simulink model "mpu6050"  (R2023b)
settings: Solver=FixedStepAuto  StartTime=0.0  StopTime=100.0  RelTol=1e-3
undefined symbols (not defined in the file): f
libraries: svdutilitieslib x1, instrumentlib x1, vrlib x1
settings Model: ExtModeTrigDuration=2  Creator=VASU  LastModifiedBy=VASU
settings OptimizationCC: EnhancedBackFolding=on  PassReuseOutputArgsAs=Individual arguments  ZeroExternalMemoryAtStartup=off  ZeroInternalMemoryAtStartup=off  MaxStackSize=64  OptimizeBlockOrder=speed  DifferentSizesBufferReuse=on  OptimizationCustomize=off  EfficientTunableParamExpr=on
settings DebuggingCC: ParameterPrecisionLossMsg=none  ParameterTunabilityLossMsg=error
settings HardwareCC: ProdBitPerPointer=32  ProdBitPerSizeT=32  ProdBitPerPtrDiffT=32  ProdLargestAtomicInteger=Long  ProdLargestAtomicFloat=Double  ProdWordSize=32  ProdHWDeviceType=ARM Compatible->ARM Cortex  UseEmbeddedCoderFeatures=off  UseSimulinkCoderFeatures=off
settings SFSimCC: MATLABDynamicMemAlloc=off
settings RTWCC: Description=Embedded Coder  SystemTargetFile=ert.tlc  HardwareBoard=ESP32-WROOM(Arduino Compatible)  TLCOptions="-aInlineSetEventsForThisBaseRateFcn=TLC_FALSE -aSuppressMultiTaskScheduler=TLC_FALSE  -aRateBasedStepFcn=0"  TemplateMakefile=ert_default_tmf  Toolchain=ESP32
settings CodeAppCC: ForceParamTrailComments=on  IgnoreCustomStorageClasses=off  OperatorAnnotations=on  SimulinkDataObjDesc=on  SFDataObjDesc=on  InsertBlockDesc=on
settings ERTTargetCC: SupportContinuousTime=on  SupportNonInlinedSFcns=on  SupportVariableSizeSignals=on  ExtModeTransport=3  ExtModeStaticAlloc=on  ExtModeAutomaticAllocSize=off  ExtModeStaticAllocSize=65536  ExtModeMexFile=ext_xcp  ExtModeIntrfLevel=Level2 - Open

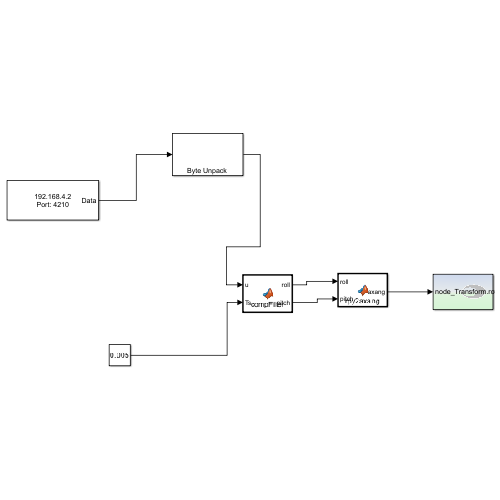
[thumbnail: Simulink's stored preview of the top-level diagram]
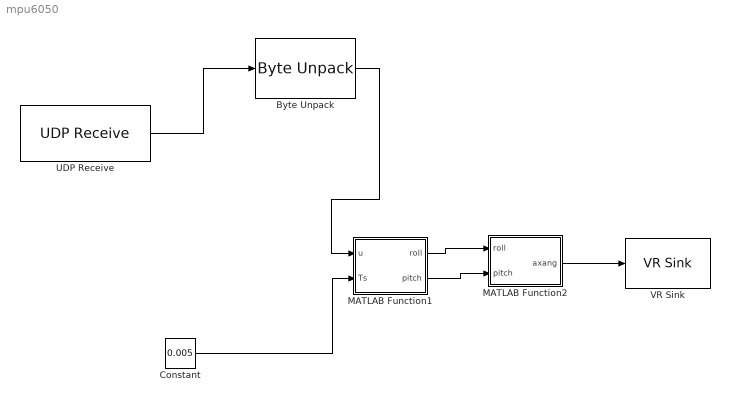
== system mpu6050 ==
  Byte Unpack : svdutilitieslib/Byte Unpack  dimensions={[6,1]}  datatypes={'single'}  byteAlign=4  blockPlatform=arduinoert
  Constant : Constant  Value=0.005  OutDataTypeStr=single
  MATLAB Function1 : MATLAB Function  TreatAsAtomicUnit=on
  MATLAB Function2 : MATLAB Function  TreatAsAtomicUnit=on
  UDP Receive : instrumentlib/UDP Receive  LocalAddress=192.168.4.2  LocalPort=4210  EnablePortSharing=on  Host=192.168.4.1  Port=4210  GetLatestData=on  DataSize=[24,1]  DataType=uint8  ASCIIFormatting=%f,  Terminator=LF  CustomTerminator=10  ByteOrder=big-endian  EnableBlockingMode=on  Timeout=10  SampleTime=0.01  SimulateUsing=Interpreted execution
  VR Sink : vrlib/VR Sink  InstantiateOnLoad=on  SampleTime=0.1  ViewEnable=on  RemoteChange=off  RemoteView=off  FieldsWritten=node_Transform.rotation.4.1.1.double  WorldFileName=C:\Users\VASU\OneDrive\Desktop\Rocketry\New folder\cansatv2\simulinkcan.x3d  AutoView=off  VideoDimensions=[]  AllowVariableSize=off
  wires:
  UDP Receive/1 -> Byte Unpack/1
  Constant/1 -> MATLAB Function1/2(Ts)
  MATLAB Function1/1(roll) -> MATLAB Function2/1(roll)
  MATLAB Function1/2(pitch) -> MATLAB Function2/2(pitch)
  MATLAB Function2/1(axang) -> VR Sink/1
  Byte Unpack/1 -> MATLAB Function1/1(u)

== matlab function mpu6050/MATLAB Function1 ==
  data: u input; roll output; Ts input; pitch output
function [roll, pitch] = compFilter(u, Ts)
% u = [ax ay az gx gy gz] (all singles from Byte Unpack)
% Ts = scalar double

ax = double(u(1));
ay = double(u(2));
az = double(u(3));
gx = double(u(4));
gy = double(u(5));
% gz = double(u(6)); % unused

Ts = double(Ts);

persistent roll_est pitch_est
if isempty(roll_est)
    roll_est = 0.0;
    pitch_est = 0.0;
end

% Accelerometer angles
roll_acc  = atan2(ay, az);
pitch_acc = atan2(-ax, sqrt(ay^2 + az^2));

% Gyro integration
roll_est  = roll_est  + gx * Ts;
pitch_est = pitch_est + gy * Ts;

% Complementary filter
alpha = 0.98;
roll  = alpha * roll_est  + (1 - alpha) * roll_acc;
pitch = alpha * pitch_est + (1 - alpha) * pitch_acc;

% Update states
roll_est  = roll;
pitch_est = pitch;
end

== matlab function mpu6050/MATLAB Function2 ==
  data: roll input; axang output; pitch input
function axang = rpy2axang(roll, pitch)
% Converts roll & pitch (radians) to axis-angle for VR Sink
% Input:  roll (rad), pitch (rad) from MPU6050 frame
% Output: [axisX axisY axisZ angle] for VR Sink

    yaw = 0;  % not measured yet

    % ---- MPU6050 → VR Sink axis mapping ----
    mapped_roll  = pitch;   % forward tilt = roll in VR
    mapped_pitch = -roll;   % right tilt = negative pitch in VR
    roll  = mapped_roll;
    pitch = mapped_pitch;
    % ----------------------------------------

    % ---- Euler (ZYX convention: yaw, pitch, roll) ----
    cy = cos(yaw/2); sy = sin(yaw/2);
    cp = cos(pitch/2); sp = sin(pitch/2);
    cr = cos(roll/2);  sr = sin(roll/2);

    % ---- Quaternion ----
    qw = cr*cp*cy + sr*sp*sy;
    qx = sr*cp*cy - cr*sp*sy;
    qy = cr*sp*cy + sr*cp*sy;
    qz = cr*cp*sy - sr*sp*cy;

    % ---- Axis-Angle ----
    angle = 2 * acos(qw);
    s = sqrt(1 - qw^2);
    if s < 1e-6
        axis = [1 0 0];
    else
        axis = [qx qy qz] / s;
    end

    axang = [axis angle];
end
